simulink model "QuadcopterPID"  (R2024b)
settings: Solver=ode23t  StartTime=0.0  StopTime=path.end_time  FixedStep=0.01  MaxStep=1e-2  RelTol=1e-3  AbsTol=1e-3
undefined symbols (not defined in the file): air_rho, battery_capacity, drone_leg, filtD_motor, filtSpd_motor, kd_motor, ki_motor, kp_motor, limit_motor, max_wind_speed, MPC_config, path, pkgSize, planedepth, qc_motor, qd_area, qd_drag, random_wind, Ts, wind_angle, wind_speed, X, Y, Z
libraries: sm_lib x78, nesl_utility x34, fl_lib x13, slpidlib x9, quadcopter_library x6, ee_lib x4, simulink x4, eeGeneralControl x1, batteryecm_lib x1
(part 1 of 4)
CloseFcn:
  | try,close(h1_quadcopter_package_delivery),end
  | clear h1_quadcopter_package_delivery
  | try,close(h2_quadcopter_package_delivery),end
  | clear h2_quadcopter_package_delivery
  | try,close(h3_quadcopter_package_delivery),end
  | clear h3_quadcopter_package_delivery
  | try,close(h4_quadcopter_package_delivery),end
  | clear h4_quadcopter_package_delivery
Description:
  | Quadcopter Package Delivery
  | Copyright 2021-2024 The MathWorks, Inc.
settings Model: VariantFading=off  Creator=tianwang  LastModifiedBy=danil
settings SolverCC: AutoScaleAbsTol=off  AlgebraicLoopSolver=TrustRegion  SolverResetMethod=Robust
settings DataIOCC: MaxDataPoints=10000  SaveOutput=off  DSMLogging=off  SaveTime=off  ReturnWorkspaceOutputs=off  TimeSaveName=timePID  SignalLoggingName=simPID
settings OptimizationCC: ReuseModelBlockBuffer=off
settings DebuggingCC: ParameterPrecisionLossMsg=none  UnconnectedInputMsg=warning  UnconnectedOutputMsg=warning  UnconnectedLineMsg=warning
settings ModelReferenceCC: EnableRefExpFcnMdlSchedulingChecks=on
settings SFSimCC: CustomCodeUndefinedFunction=UseInterfaceOnly
settings RTWCC: GPUComputeCapability=3.5  DLArmComputeVersion=19.05
settings SimscapeCC: ExplicitSolverDiagnosticOptions=none  SimscapeLogSimulationStatistics=on  SimscapeLogToSDI=on  SimscapeLogName=simlog_quadcopter_package_delivery  SimscapeLogLimitData=off  SimscapeLogDataHistory=50000
settings DiagnosticsConfigSet: SimMechanicsConflictingReferenceFrames=none  SimMechanicsRigidlyBoundBlock=none
settings ExplorerConfigSet: InternalSimMechanicsExplorerSettings="<ExplorerConfiguration><canonicalview>default</canonicalview><AnimationSetting><BasePlaybackSpeed>1.0</BasePlaybackSpeed><PlaybackSpeedFactor>1.0</PlaybackSpeedFactor></AnimationSetting><TilePanel><TileInfo><Tiles Columns=\"2\" Count=\"4\" Rows=\"2\"><Column Weight=\"0.5108\"/><Column Weight=\"0.4892\"/><Row Weight=\"0.4948\"/><Row Weight=\"0.5052\"/><Tile Height=\"1\" Width=\"1\" X=\"0\" Y=\"0\"/><Tile Height=\"1\" Width=\"1\" X=\"0\" Y=\"1\"/><Tile Height=\"1\" Width=\"1\" X=\"1\" Y=\"0\"/><Tile Height=\"1\" Width=\"1\" X=\"1\" Y=\"1\"/></Tiles></TileInfo><SceneInfo><SceneViewer><BGColor><R>1</R><G>1</G><B>1</B></BGColor><Camera><DoPerspective>off</DoPerspective><Position><X>-3.99027915045383441</X><Y>0.687031223743990171</Y><Z>68.9498413117964901</Z></Position><Center><X>-3.99027915045383441</X><Y>0.687031223743990171</Y><Z>3.00000062058594352</Z></Center><Up><X>0</X><Y>1</Y><Z>-0</Z></Up><ViewLimDist>1</ViewLimDist><YLim>5.31135561676258483</YLim><XLim>8.87109395565665793</XLim></Camera></SceneViewer><SceneViewer><BGColor><R>1</R><G>1</G><B>1</B></BGColor><Camera><DoPerspective>on</DoPerspective><Position><X>9.88101233232043086</X><Y>10.0748186090521319</Y><Z>2.02141500533963869</Z></Position><Center><X>9.88101233232043086</X><Y>10.0748186090521319</Y><Z>1.02141500533963869</Z></Center><Up><X>0</X><Y>1</Y><Z>0</Z></Up><ViewLimDist>1</ViewLimDist><YLim>0.466307658154998583</YLim><XLim>0.762607315940987296</XLim></Camera></SceneViewer><SceneViewer><BGColor><R>0.200000002980232239</R><G>0.60000002384185791</G><B>1</B></BGColor><Camera><DoPerspective>on</DoPerspective><Position><X>11.5</X><Y>8.5</Y><Z>1.14000000000000012</Z></Position><Center><X>10</X><Y>10</Y><Z>0.140000000000000013</Z></Center><Up><X>0</X><Y>0</Y><Z>1</Z></Up><ViewLimDist>1</ViewLimDist><YLim>0.466307658154998583</YLim><XLim>0.745761538396823909</XLim></Camera></SceneViewer><SceneViewer><BGColor><R>1</R><G>1</G><B>1</B></BGColor><Camera><DoPerspective>on</DoPerspective><Position><X>10.3810123323204309</X><Y>9.07481860905213189</Y><Z>2.02141500533963869</Z></Position><Center><X>10.0476789989870969</X><Y>9.74148527571879796</Y><Z>1.35474833867297195</Z></Center><Up><X>-0.298142396999971915</X><Y>0.596284793999944052</Y><Z>0.745355992499929787</Z></Up><ViewLimDist>1</ViewLimDist><YLim>0.466307658154998583</YLim><XLim>0.730224839680223559</XLim></Camera></SceneViewer></SceneInfo></TilePanel><MechEditorPanel><Cameras><Camera><Id>Camera1</Id><Value><Name>FixO Top</Name><NativeCamera><PositionTrackingFeature>Quadcopter.Camera.Cam_FixO_Top.R</PositionTrackingFeature><CenterTrackingFeature>Quadcopter.Camera.Cam_FixO_Top.R</CenterTrackingFeature><UpVectorTrackingFeature>Quadcopter.Camera.Cam_FixO_Top.R</UpVectorTrackingFeature><CenterTrackingOrigin>off</CenterTrackingOrigin><CenterTrackingDirection>+X</CenterTrackingDirection><UpVectorTrackingDirection>+Y</UpVectorTrackingDirection></NativeCamera></Value></Camera><Camera><Id>Camera2</Id><Value><Name>FixO L</Name><NativeCamera><PositionTrackingFeature>Quadcopter.Camera.Cam_FixO_L.R</PositionTrackingFeature><CenterTrackingFeature>Quadcopter.Camera.Cam_FixO_L.R</CenterTrackingFeature><UpVectorTrackingFeature>Quadcopter.Camera.Cam_FixO_L.R</UpVectorTrackingFeature><CenterTrackingOrigin>off</CenterTrackingOrigin><CenterTrackingDirection>+X</CenterTrackingDirection><UpVectorTrackingDirection>+Z</UpVectorTrackingDirection></NativeCamera></Value></Camera><Camera><Id>Camera3</Id><Value><Name>FixO F</Name><NativeCamera><PositionTrackingFeature>Quadcopter.Camera.Cam_FixO_F.R</PositionTrackingFeature><CenterTrackingFeature>Quadcopter.Camera.Cam_FixO_F.R</CenterTrackingFeature><UpVectorTrackingFeature>Quadcopter.Camera.Cam_FixO_F.R</UpVectorTrackingFeature><CenterTrackingOrigin>off</CenterTrackingOrigin><CenterTrackingDirection>+X</CenterTrackingDirection><UpVectorTrackingDirection>+Z</UpVectorTrackingDirection></NativeCamera></Value></Camera><Camera><Id>Camera4</Id><Value><Name>FixO UFL</Name><NativeCamera><PositionTrackingFeature>Quadcopter.Camera.Cam_FixO_UFL.R</PositionTrackingFeature><CenterTrackingFeature>Quadcopter.Camera.Cam_FixO_UFL.R</CenterTrackingFeature><UpVectorTrackingFeature>Quadcopter.Camera.Cam_FixO_UFL.R</UpVectorTrackingFeature><CenterTrackingOrigin>off</CenterTrackingOrigin><CenterTrackingDirection>+X</CenterTrackingDirection><UpVectorTrackingDirection>+Z</UpVectorTrackingDirection></NativeCamera></Value></Camera><Camera><Id>Camera5</Id><Value><Name>Track_Target</Name><NativeCamera><PositionTrackingFeature>Quadcopter.Camera.Cam_Target.R</PositionTrackingFeature><CenterTrackingFeature>Quadcopter.Camera.Transform_Target.F</CenterTrackingFeature><UpVectorTrackingFeature>Quadcopter.Camera.Transform_Target.F</UpVectorTrackingFeature><CenterTrackingOrigin>on</CenterTrackingOrigin><UpVectorTrackingDirection>+Z</UpVectorTrackingDirection></NativeCamera></Value></Camera><Camera><Id>Camera6</Id><Value><Name>Track Body Forward</Name><NativeCamera><PositionTrackingFeature>Quadcopter.Body.Body.Cam_Body_Front.R</PositionTrackingFeature><CenterTrackingFeature>Quadcopter.Body.Body.Cam_Body_Front.R</CenterTrackingFeature><UpVectorTrackingFeature>Quadcopter.Body.Body.Cam_Body_Front.R</UpVectorTrackingFeature><CenterTrackingOrigin>off</CenterTrackingOrigin><CenterTrackingDirection>+X</CenterTrackingDirection><UpVectorTrackingDirection>+Z</UpVectorTrackingDirection></NativeCamera></Value></Camera></Cameras><GfxPanelCameraMap><MapElement CameraMLId=\"Camera1\" GfxPanelIndex=\"1\"/><MapElement CameraMLId=\"Camera5\" GfxPanelIndex=\"2\"/><MapElement CameraMLId=\"Camera4\" GfxPanelIndex=\"3\"/></GfxPanelCameraMap><VideoCreator><PlaybackSpeedRatio>1.0</PlaybackSpeedRatio><FrameRate>60</FrameRate><VideoFormat>MPEG-4</VideoFormat><FrameSize>[1920 1080]</FrameSize></VideoCreator></MechEditorPanel></ExplorerConfiguration>"

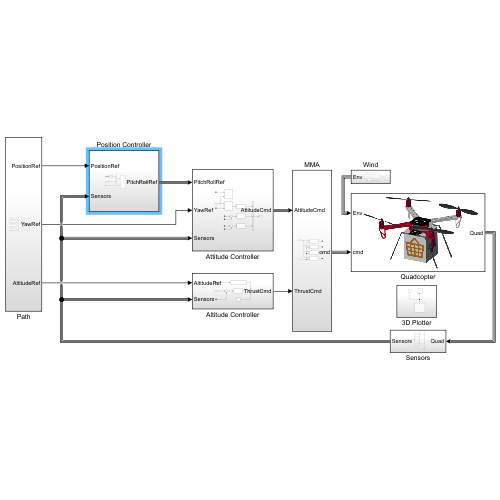
[thumbnail: Simulink's stored preview of the top-level diagram]
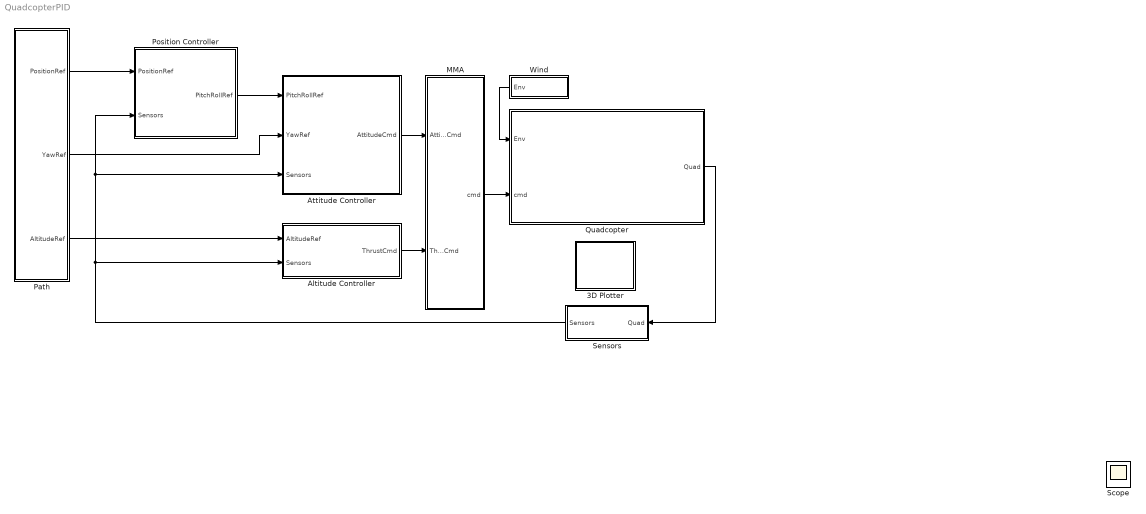
== system QuadcopterPID ==
  3D Plotter : Subsystem
  Altitude Controller : Subsystem
  Attitude Controller : Subsystem
  MMA : Subsystem
  Path : Subsystem
  Position Controller : Subsystem
  Quadcopter : Subsystem
      mask Display:
      | % image('quadcopter_body_arms_load.png');
      | image('quadcopter_body_arms_load_basket.png');
  Sensors : Subsystem
  Wind : Subsystem
  Scope : Scope
  wires:
  Wind/1(Env) -> Quadcopter/1(Env)
  Path/1(PositionRef) -> Position Controller/1(PositionRef)
  Altitude Controller/1(ThrustCmd) -> MMA/2(ThrustCmd)
  MMA/1(cmd) -> Quadcopter/2(cmd)
  Sensors/1(Sensors) -> Position Controller/2(Sensors), Attitude Controller/3(Sensors), Altitude Controller/2(Sensors)
  Path/2(YawRef) -> Attitude Controller/2(YawRef)
  Attitude Controller/1(AttitudeCmd) -> MMA/1(AttitudeCmd)
  Position Controller/1(PitchRollRef) -> Attitude Controller/1(PitchRollRef)
  Path/3(AltitudeRef) -> Altitude Controller/1(AltitudeRef)
  Quadcopter/1(Quad) -> Sensors/1(Quad)

== system QuadcopterPID/3D Plotter ==
  Path : Subsystem
      settings: PortSchema="{\"entries\":[{\"content\":{\"sides\":[{\"content\":{},\"type\":\"ConnectorPlacement.EquallySpacedRectSide\",\"uuid\":\"a37decf6-7c95-4e74-978f-accab4815bca\"},{\"content\":{\"side\":\"RIGHT\"},\"type\":\"ConnectorPlacement.EquallySpacedRectSide\",\"uuid\":\"1290ed2a-5cda-4ac5-b3d1-08d972a37bb4\"},{\"content\":{\"side\":\"TOP\"},\"type\":\"ConnectorPlacement.EquallySpacedRectSide\",\"uuid\":\"57cc8f3c-04dd-443b-a82e-0db9ef1adeeb\"},{\"content\":{\"connectorIds\":[\"RConn1\"],\"side\":\"BOTTOM\"},\"type\":\"ConnectorPlacement.EquallySpacedRectSide\",\"uuid\":\"a98ac24c-8795-4aa4-8cf5-242b040624e5\"}]},\"type\":\"ConnectorPlacement.EquallySpacedConnector\",\"uuid\":\"16016d0d-0355-4838-b6b7-987ac63207fe\"}],\"packageUris\":[\"http://schema.mathworks.com/mf0/Connector/R2020b\"],\"version\":\"1.0\"}"
  Solver Configuration : nesl_utility/Solver Configuration  PhysicalDomain=network_engine_domain  SubClassName=solver  LeftPortType=input  RightPortType=generic  Tones=[]  Harmonics=[]  SimulateNoise=off  Profile=off  UseLocalSampling=off  EnableSwitchedLinearOptims=on  FrequencyDomain=off  UseCCode=off  RelTol=0.001  AbsTol=0.001  MinStep=1e-09  ToWorkspace=off  RevertToSquareIcSolve=off  NumHomotopyIterations=100  PhasorMode=off  PhasorModeNumHarmonics=1  ConsistencySolver=NEWTON_XTOL_AFTER_FTOL  IndexReductionMethod=DerivativeReplacement  DoDC=off  ResidualTolerance=1e-09  ConsistencyTolSource=GLOBAL  ConsistencyAbsTol=0.001  ConsistencyRelTol=0.001  ConsistencyTolFactor=0.001  UseLocalSolver=off  LocalSolverChoice=NE_BACKWARD_EULER_ADVANCER  ResolveIndetEquations=on  FunctionEvalNumThread=1  LocalSolverSampleTime=0.001  DoFixedCost=off  MaxNonlinIter=3  MaxModeIter=2  ComputeImpulses=off  ImpulseIterations=2  LinearAlgebra=auto  LinearAlgebraNumThread=0  EquationFormulation=NE_TIME_EF  DelaysMemoryBudget=1024  AutomaticFiltering=on  FilteringTimeConstant=0.001  PartitionStorageMethod=AS_NEEDED  PartitionMemoryBudget=1024  PartitionMethod=ROBUST  MultibodyUseLocalSolver=off  MultibodyLocalSolverChoice=ODE1  MultibodyLocalSolverSampleTime=0.001
  World Frame : sm_lib/Frames and Transforms/World Frame
  connections:
  World Frame/RConn1 -- Solver Configuration/RConn1 -- Path/RConn1

== system QuadcopterPID/Altitude Controller ==
  AltitudeRef : Inport
  BusElementIn : Inport  Port=2  PortName=Sensors  Element=Position.pz
  BusElementIn1 : Inport  Port=2  PortName=Sensors  Element=LoadStatus
  Constant : Constant  Value=4500
  Control Thrust : slpidlib/PID Controller  Controller=PID  Form=Parallel  TimeDomain=Discrete-time  UseExternalTs=off  SampleTime=-1  IntegratorMethod=Forward Euler  FilterMethod=Forward Euler  ControllerParametersSource=internal  P=2500  I=800  UseKiTs=off  D=3200  UseExternalDerivativeSource=off  N=100  UseFilter=on  TunerSelectOption=Transfer Function Based (PID Tuner App)  ZeroCross=off  InitialConditionSource=internal  InitialConditionForIntegrator=0  InitialConditionForFilter=0  DifferentiatorICPrevScaledInput=0  ExternalReset=none  TrackingMode=off  Kt=1  LimitOutput=on  SatLimitsSource=internal  UpperSaturationLimit=85695  LowerSaturationLimit=-85695  LinearizeAsGain=on  AntiWindupMode=none  Kb=1  LimitIntegrator=off  UpperIntegratorSaturationLimit=inf  LowerIntegratorSaturationLimit=-inf  POutMin=[]  POutMax=[]  IOutMin=[]  IOutMax=[]  DOutMin=[]  DOutMax=[]  NOutMin=[]  NOutMax=[]  SumOutMin=[]  SumOutMax=[]  SaturationOutMin=[]  SaturationOutMax=[]  PParamMin=[]  PParamMax=[]  IParamMin=[]  IParamMax=[]  DParamMin=[]  DParamMax=[]  NParamMin=[]  NParamMax=[]  KbParamMin=[]  KbParamMax=[]  KtParamMin=[]  KtParamMax=[]  KbOutMin=[]  KbOutMax=[]  KtOutMin=[]  KtOutMax=[]  IntegratorOutMin=[]  IntegratorOutMax=[]  FilterOutMin=[]  FilterOutMax=[]  SumI1OutMin=[]  SumI1OutMax=[]  SumI2OutMin=[]  SumI2OutMax=[]  SumI3OutMin=[]  SumI3OutMax=[]  SumI4OutMin=[]  SumI4OutMax=[]  SumDOutMin=[]  SumDOutMax=[]  DifferentiatorOutMin=[]  DifferentiatorOutMax=[]  FilterDiffOutCoefMin=[]  FilterDiffOutCoefMax=[]  ReciprocalOutMin=[]  ReciprocalOutMax=[]  SumDenOutMin=[]  SumDenOutMax=[]  SumNumOutMin=[]  SumNumOutMax=[]  DivideOutMin=[]  DivideOutMax=[]  UdiffTsProdOutMin=[]  UdiffTsProdOutMax=[]  NTsProdOutMin=[]  NTsProdOutMax=[]  UintegralTsProdOutMin=[]  UintegralTsProdOutMax=[]  UngainTsProdOutMin=[]  UngainTsProdOutMax=[]  ClampingZeroOutDataTypeStr=Inherit: Inherit via back propagation  ClampingZeroOutMin=[]  ClampingZeroOutMax=[]  FilterDenConstantOutDataTypeStr=Inherit: Inherit via back propagation  FilterDenConstantOutMin=[]  FilterDenConstantOutMax=[]  PCopyOutDataTypeStr=Inherit: Inherit via back propagation  PCopyOutMin=[]  PCopyOutMax=[]  NCopyOutDataTypeStr=Inherit: Inherit via back propagation  NCopyOutMin=[]  NCopyOutMax=[]  IntegratorContinuousStateAttributes=''  IntegratorStateMustResolveToSignalObject=off  IntegratorRTWStateStorageClass=Auto  FilterContinuousStateAttributes=''  FilterStateMustResolveToSignalObject=off  FilterRTWStateStorageClass=Auto  ParallelPVariant=InternalParameters  IdealPVariant=Disabled  IVariant=InternalParameters  DVariant=InternalParameters  IntegratorVariant=Discrete  SatVariant=Enabled  AWVariant=Passthrough  PCopyVariant=Disabled  TRVariant=Disabled  FdbkBlocksVariant=Forward  IdealPFdbkVariant=Disabled  SatFdbkVariant=Disabled  DerivativeFilterVariant=ForwardEulerFilter  NVariant=InternalParameters  NCopyVariant=Disabled  FilterICVariant=InternalICsFilter  IntegratorICVariant=InternalICs  ExternalResetVariant=Disabled  TRSumVariant=Passthrough  SumFdbkVariant=Disabled  SumVariant=Sum_PID  TsampFilterVariant=InternalTs  TsampNgainVariant=Passthrough  TsampIntegralVariant=Disabled_SignalSpec  ExternalSaturationOutDataTypeStr=Inherit: Same as second input  DerivativeSourceVariant=ErrorSignal  PreIntVariant=InternalPreInt
  Subsystem : Subsystem
  Sum : Sum  Inputs=+++
  Sum1 : Sum  Inputs=|+-
  ThrustCmd : Outport
  wires:
  Sum1/1 -> Control Thrust/1
  BusElementIn/1 -> Sum1/2
  AltitudeRef/1 -> Sum1/1
  Sum/1 -> ThrustCmd/1
  Constant/1 -> Sum/3  "Drone Bias"
  Control Thrust/1 -> Sum/2
  Subsystem/1(Load Bias) -> Sum/1
  BusElementIn1/1 -> Subsystem/1(Load Status)

== system QuadcopterPID/Attitude Controller ==
  Bus Element In1 : Inport  PortName=PitchRollRef
  Bus Element In4 : Inport  PortName=PitchRollRef  Element=pitch
  Bus Element In5 : Inport  PortName=PitchRollRef  Element=roll
  YawRef : Inport  Port=2
  BusElementIn2 : Inport  Port=3  PortName=Sensors  Element=Attitude.roll
  BusElementIn : Inport  Port=3  PortName=Sensors  Element=Attitude.yaw
  BusElementIn1 : Inport  Port=3  PortName=Sensors  Element=Attitude.pitch
  Angle Difference : Subsystem
  Bus Creator : BusCreator  Inputs=3
  Control Pitch : slpidlib/PID Controller  Controller=PID  Form=Parallel  TimeDomain=Discrete-time  UseExternalTs=off  SampleTime=-1  IntegratorMethod=Forward Euler  FilterMethod=Forward Euler  ControllerParametersSource=internal  P=2200  I=3500  UseKiTs=off  D=500  UseExternalDerivativeSource=off  N=100  UseFilter=on  TunerSelectOption=Transfer Function Based (PID Tuner App)  InitialConditionSource=internal  InitialConditionForIntegrator=0  InitialConditionForFilter=0  DifferentiatorICPrevScaledInput=0  ExternalReset=none  TrackingMode=off  Kt=1  LimitOutput=on  SatLimitsSource=internal  UpperSaturationLimit=800  LowerSaturationLimit=-800  LinearizeAsGain=on  AntiWindupMode=clamping  Kb=1  LimitIntegrator=off  UpperIntegratorSaturationLimit=inf  LowerIntegratorSaturationLimit=-inf  POutMin=[]  POutMax=[]  IOutMin=[]  IOutMax=[]  DOutMin=[]  DOutMax=[]  NOutMin=[]  NOutMax=[]  SumOutMin=[]  SumOutMax=[]  SaturationOutMin=[]  SaturationOutMax=[]  PParamMin=[]  PParamMax=[]  IParamMin=[]  IParamMax=[]  DParamMin=[]  DParamMax=[]  NParamMin=[]  NParamMax=[]  KbParamMin=[]  KbParamMax=[]  KtParamMin=[]  KtParamMax=[]  KbOutMin=[]  KbOutMax=[]  KtOutMin=[]  KtOutMax=[]  IntegratorOutMin=[]  IntegratorOutMax=[]  FilterOutMin=[]  FilterOutMax=[]  SumI1OutMin=[]  SumI1OutMax=[]  SumI2OutMin=[]  SumI2OutMax=[]  SumI3OutMin=[]  SumI3OutMax=[]  SumI4OutMin=[]  SumI4OutMax=[]  SumDOutMin=[]  SumDOutMax=[]  DifferentiatorOutMin=[]  DifferentiatorOutMax=[]  FilterDiffOutCoefMin=[]  FilterDiffOutCoefMax=[]  ReciprocalOutMin=[]  ReciprocalOutMax=[]  SumDenOutMin=[]  SumDenOutMax=[]  SumNumOutMin=[]  SumNumOutMax=[]  DivideOutMin=[]  DivideOutMax=[]  UdiffTsProdOutMin=[]  UdiffTsProdOutMax=[]  NTsProdOutMin=[]  NTsProdOutMax=[]  UintegralTsProdOutMin=[]  UintegralTsProdOutMax=[]  UngainTsProdOutMin=[]  UngainTsProdOutMax=[]  ClampingZeroOutDataTypeStr=Inherit: Inherit via back propagation  ClampingZeroOutMin=[]  ClampingZeroOutMax=[]  FilterDenConstantOutDataTypeStr=Inherit: Inherit via back propagation  FilterDenConstantOutMin=[]  FilterDenConstantOutMax=[]  PCopyOutDataTypeStr=Inherit: Inherit via back propagation  PCopyOutMin=[]  PCopyOutMax=[]  NCopyOutDataTypeStr=Inherit: Inherit via back propagation  NCopyOutMin=[]  NCopyOutMax=[]  IntegratorContinuousStateAttributes=''  IntegratorStateMustResolveToSignalObject=off  IntegratorRTWStateStorageClass=Auto  FilterContinuousStateAttributes=''  FilterStateMustResolveToSignalObject=off  FilterRTWStateStorageClass=Auto  ParallelPVariant=InternalParameters  IdealPVariant=Disabled  IVariant=InternalParameters  DVariant=InternalParameters  IntegratorVariant=Discrete  SatVariant=Enabled  AWVariant=DiscClampingParallel  PCopyVariant=Disabled  TRVariant=Disabled  FdbkBlocksVariant=Forward  IdealPFdbkVariant=Disabled  SatFdbkVariant=Disabled  DerivativeFilterVariant=ForwardEulerFilter  NVariant=InternalParameters  NCopyVariant=Disabled  FilterICVariant=InternalICsFilter  IntegratorICVariant=InternalICs  ExternalResetVariant=Disabled  TRSumVariant=Passthrough  SumFdbkVariant=Disabled  SumVariant=Sum_PID  TsampFilterVariant=InternalTs  TsampNgainVariant=Passthrough  TsampIntegralVariant=Disabled_SignalSpec  ExternalSaturationOutDataTypeStr=Inherit: Same as second input  DerivativeSourceVariant=ErrorSignal  PreIntVariant=InternalPreInt
  Control Roll : slpidlib/PID Controller  Controller=PID  Form=Parallel  TimeDomain=Discrete-time  UseExternalTs=off  SampleTime=-1  IntegratorMethod=Forward Euler  FilterMethod=Forward Euler  ControllerParametersSource=internal  P=2200  I=3500  UseKiTs=off  D=500  UseExternalDerivativeSource=off  N=100  UseFilter=on  TunerSelectOption=Transfer Function Based (PID Tuner App)  InitialConditionSource=internal  InitialConditionForIntegrator=0  InitialConditionForFilter=0  DifferentiatorICPrevScaledInput=0  ExternalReset=none  TrackingMode=off  Kt=1  LimitOutput=on  SatLimitsSource=internal  UpperSaturationLimit=800  LowerSaturationLimit=-800  LinearizeAsGain=on  AntiWindupMode=clamping  Kb=1  LimitIntegrator=off  UpperIntegratorSaturationLimit=inf  LowerIntegratorSaturationLimit=-inf  POutMin=[]  POutMax=[]  IOutMin=[]  IOutMax=[]  DOutMin=[]  DOutMax=[]  NOutMin=[]  NOutMax=[]  SumOutMin=[]  SumOutMax=[]  SaturationOutMin=[]  SaturationOutMax=[]  PParamMin=[]  PParamMax=[]  IParamMin=[]  IParamMax=[]  DParamMin=[]  DParamMax=[]  NParamMin=[]  NParamMax=[]  KbParamMin=[]  KbParamMax=[]  KtParamMin=[]  KtParamMax=[]  KbOutMin=[]  KbOutMax=[]  KtOutMin=[]  KtOutMax=[]  IntegratorOutMin=[]  IntegratorOutMax=[]  FilterOutMin=[]  FilterOutMax=[]  SumI1OutMin=[]  SumI1OutMax=[]  SumI2OutMin=[]  SumI2OutMax=[]  SumI3OutMin=[]  SumI3OutMax=[]  SumI4OutMin=[]  SumI4OutMax=[]  SumDOutMin=[]  SumDOutMax=[]  DifferentiatorOutMin=[]  DifferentiatorOutMax=[]  FilterDiffOutCoefMin=[]  FilterDiffOutCoefMax=[]  ReciprocalOutMin=[]  ReciprocalOutMax=[]  SumDenOutMin=[]  SumDenOutMax=[]  SumNumOutMin=[]  SumNumOutMax=[]  DivideOutMin=[]  DivideOutMax=[]  UdiffTsProdOutMin=[]  UdiffTsProdOutMax=[]  NTsProdOutMin=[]  NTsProdOutMax=[]  UintegralTsProdOutMin=[]  UintegralTsProdOutMax=[]  UngainTsProdOutMin=[]  UngainTsProdOutMax=[]  ClampingZeroOutDataTypeStr=Inherit: Inherit via back propagation  ClampingZeroOutMin=[]  ClampingZeroOutMax=[]  FilterDenConstantOutDataTypeStr=Inherit: Inherit via back propagation  FilterDenConstantOutMin=[]  FilterDenConstantOutMax=[]  PCopyOutDataTypeStr=Inherit: Inherit via back propagation  PCopyOutMin=[]  PCopyOutMax=[]  NCopyOutDataTypeStr=Inherit: Inherit via back propagation  NCopyOutMin=[]  NCopyOutMax=[]  IntegratorContinuousStateAttributes=''  IntegratorStateMustResolveToSignalObject=off  IntegratorRTWStateStorageClass=Auto  FilterContinuousStateAttributes=''  FilterStateMustResolveToSignalObject=off  FilterRTWStateStorageClass=Auto  ParallelPVariant=InternalParameters  IdealPVariant=Disabled  IVariant=InternalParameters  DVariant=InternalParameters  IntegratorVariant=Discrete  SatVariant=Enabled  AWVariant=DiscClampingParallel  PCopyVariant=Disabled  TRVariant=Disabled  FdbkBlocksVariant=Forward  IdealPFdbkVariant=Disabled  SatFdbkVariant=Disabled  DerivativeFilterVariant=ForwardEulerFilter  NVariant=InternalParameters  NCopyVariant=Disabled  FilterICVariant=InternalICsFilter  IntegratorICVariant=InternalICs  ExternalResetVariant=Disabled  TRSumVariant=Passthrough  SumFdbkVariant=Disabled  SumVariant=Sum_PID  TsampFilterVariant=InternalTs  TsampNgainVariant=Passthrough  TsampIntegralVariant=Disabled_SignalSpec  ExternalSaturationOutDataTypeStr=Inherit: Same as second input  DerivativeSourceVariant=ErrorSignal  PreIntVariant=InternalPreInt
  Control Yaw : slpidlib/PID Controller  Controller=PID  Form=Parallel  TimeDomain=Discrete-time  UseExternalTs=off  SampleTime=-1  IntegratorMethod=Forward Euler  FilterMethod=Forward Euler  ControllerParametersSource=internal  P=3000  I=1200  UseKiTs=off  D=0  UseExternalDerivativeSource=off  N=100  UseFilter=on  TunerSelectOption=Transfer Function Based (PID Tuner App)  InitialConditionSource=internal  InitialConditionForIntegrator=0  InitialConditionForFilter=0  DifferentiatorICPrevScaledInput=0  ExternalReset=none  TrackingMode=off  Kt=1  LimitOutput=on  SatLimitsSource=internal  UpperSaturationLimit=400  LowerSaturationLimit=-400  LinearizeAsGain=on  AntiWindupMode=clamping  Kb=1  LimitIntegrator=off  UpperIntegratorSaturationLimit=inf  LowerIntegratorSaturationLimit=-inf  POutMin=[]  POutMax=[]  IOutMin=[]  IOutMax=[]  DOutMin=[]  DOutMax=[]  NOutMin=[]  NOutMax=[]  SumOutMin=[]  SumOutMax=[]  SaturationOutMin=[]  SaturationOutMax=[]  PParamMin=[]  PParamMax=[]  IParamMin=[]  IParamMax=[]  DParamMin=[]  DParamMax=[]  NParamMin=[]  NParamMax=[]  KbParamMin=[]  KbParamMax=[]  KtParamMin=[]  KtParamMax=[]  KbOutMin=[]  KbOutMax=[]  KtOutMin=[]  KtOutMax=[]  IntegratorOutMin=[]  IntegratorOutMax=[]  FilterOutMin=[]  FilterOutMax=[]  SumI1OutMin=[]  SumI1OutMax=[]  SumI2OutMin=[]  SumI2OutMax=[]  SumI3OutMin=[]  SumI3OutMax=[]  SumI4OutMin=[]  SumI4OutMax=[]  SumDOutMin=[]  SumDOutMax=[]  DifferentiatorOutMin=[]  DifferentiatorOutMax=[]  FilterDiffOutCoefMin=[]  FilterDiffOutCoefMax=[]  ReciprocalOutMin=[]  ReciprocalOutMax=[]  SumDenOutMin=[]  SumDenOutMax=[]  SumNumOutMin=[]  SumNumOutMax=[]  DivideOutMin=[]  DivideOutMax=[]  UdiffTsProdOutMin=[]  UdiffTsProdOutMax=[]  NTsProdOutMin=[]  NTsProdOutMax=[]  UintegralTsProdOutMin=[]  UintegralTsProdOutMax=[]  UngainTsProdOutMin=[]  UngainTsProdOutMax=[]  ClampingZeroOutDataTypeStr=Inherit: Inherit via back propagation  ClampingZeroOutMin=[]  ClampingZeroOutMax=[]  FilterDenConstantOutDataTypeStr=Inherit: Inherit via back propagation  FilterDenConstantOutMin=[]  FilterDenConstantOutMax=[]  PCopyOutDataTypeStr=Inherit: Inherit via back propagation  PCopyOutMin=[]  PCopyOutMax=[]  NCopyOutDataTypeStr=Inherit: Inherit via back propagation  NCopyOutMin=[]  NCopyOutMax=[]  IntegratorContinuousStateAttributes=''  IntegratorStateMustResolveToSignalObject=off  IntegratorRTWStateStorageClass=Auto  FilterContinuousStateAttributes=''  FilterStateMustResolveToSignalObject=off  FilterRTWStateStorageClass=Auto  ParallelPVariant=InternalParameters  IdealPVariant=Disabled  IVariant=InternalParameters  DVariant=InternalParameters  IntegratorVariant=Discrete  SatVariant=Enabled  AWVariant=DiscClampingParallel  PCopyVariant=Disabled  TRVariant=Disabled  FdbkBlocksVariant=Forward  IdealPFdbkVariant=Disabled  SatFdbkVariant=Disabled  DerivativeFilterVariant=ForwardEulerFilter  NVariant=InternalParameters  NCopyVariant=Disabled  FilterICVariant=InternalICsFilter  IntegratorICVariant=InternalICs  ExternalResetVariant=Disabled  TRSumVariant=Passthrough  SumFdbkVariant=Disabled  SumVariant=Sum_PID  TsampFilterVariant=InternalTs  TsampNgainVariant=Passthrough  TsampIntegralVariant=Disabled_SignalSpec  ExternalSaturationOutDataTypeStr=Inherit: Same as second input  DerivativeSourceVariant=ErrorSignal  PreIntVariant=InternalPreInt
  Data Inspector Plotter : Subsystem
  Sum1 : Sum  Inputs=|+-
  Sum2 : Sum  Inputs=|+-
  AttitudeCmd : Outport
  wires:
  BusElementIn2/1 -> Sum2/2
  Bus Creator/1 -> AttitudeCmd/1
  Bus Element In4/1 -> Sum1/1
  Bus Element In5/1 -> Sum2/1
  YawRef/1 -> Data Inspector Plotter/2(YawRef), Angle Difference/1(YawRef)
  BusElementIn/1 -> Angle Difference/2(Yaw)
  BusElementIn1/1 -> Sum1/2
  Angle Difference/1(Diff) -> Control Yaw/1
  Control Yaw/1 -> Bus Creator/1  "yawCmd"
  Sum1/1 -> Control Pitch/1
  Control Pitch/1 -> Bus Creator/2  "pitchCmd"
  Sum2/1 -> Control Roll/1
  Control Roll/1 -> Bus Creator/3  "rollCmd"
  Bus Element In1/1 -> Data Inspector Plotter/1(PitchRollRef)

== system QuadcopterPID/MMA ==
  AttitudeCmd : Inport
  ThrustCmd : Inport  Port=2
  Calculate w1 : Subsystem
  Calculate w2 : Subsystem
  Calculate w3 : Subsystem
  Calculate w4 : Subsystem
  Bus Element Out : Outport  PortName=cmd  Element=w1
  Bus Element Out1 : Outport  PortName=cmd  Element=w2
  Bus Element Out2 : Outport  PortName=cmd  Element=w3
  Bus Element Out3 : Outport  PortName=cmd  Element=w4
  wires:
  Calculate w1/1(w1) -> Bus Element Out/1
  Calculate w4/1(w4) -> Bus Element Out3/1
  Calculate w3/1(w3) -> Bus Element Out2/1
  Calculate w2/1(w2) -> Bus Element Out1/1
  AttitudeCmd/1 -> Calculate w4/1(AttitudeCmd), Calculate w3/1(AttitudeCmd), Calculate w2/1(AttitudeCmd), Calculate w1/1(AttitudeCmd)
  ThrustCmd/1 -> Calculate w4/2(ThrustCmd), Calculate w3/2(ThrustCmd), Calculate w2/2(ThrustCmd), Calculate w1/2(ThrustCmd)

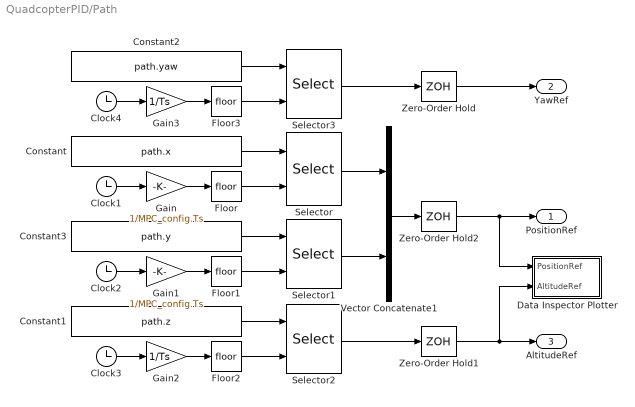
== system QuadcopterPID/Path ==
  Clock{1..4} (4 alike) : Clock
  Constant : Constant  Value=path.x
  Constant1 : Constant  Value=path.z
  Constant2 : Constant  Value=path.yaw
  Constant3 : Constant  Value=path.y
  Data Inspector Plotter : Subsystem
      settings: PortSchema="{\"entries\":[{\"content\":{\"sides\":[{\"content\":{},\"type\":\"ConnectorPlacement.EquallySpacedRectSide\",\"uuid\":\"0f496bf2-b2b6-4bd2-9425-cb84c143776b\"},{\"content\":{\"side\":\"RIGHT\"},\"type\":\"ConnectorPlacement.EquallySpacedRectSide\",\"uuid\":\"68946bc1-57df-4a88-8dd1-ab10ea4e76e5\"},{\"content\":{\"side\":\"TOP\"},\"type\":\"ConnectorPlacement.EquallySpacedRectSide\",\"uuid\":\"57e381a0-7f21-49e7-882a-f855c26e7315\"},{\"content\":{\"connectorIds\":[\"In1\",\"In2\"],\"side\":\"BOTTOM\"},\"type\":\"ConnectorPlacement.EquallySpacedRectSide\",\"uuid\":\"a1114455-6af3-4814-9eeb-f18f60502d18\"}]},\"type\":\"ConnectorPlacement.EquallySpacedConnector\",\"uuid\":\"8716bf71-a1b6-4b1a-bd8c-297568339aba\"}],\"packageUris\":[\"http://schema.mathworks.com/mf0/Connector/R2020b\"],\"version\":\"1.0\"}"
  Floor{,1..3} (4 alike) : Rounding
  Gain : Gain  Gain=1/MPC_config.Ts
  Gain1 : Gain  Gain=1/MPC_config.Ts
  Gain2 : Gain  Gain=1/Ts
  Gain3 : Gain  Gain=1/Ts
  Selector : Selector  IndexMode=Zero-based  InputPortWidth=size(path.x,2)  IndexOptions=Index vector (port)  Indices=[1 3]  OutputSizes=MPC_config.N
  Selector1 : Selector  IndexMode=Zero-based  InputPortWidth=size(path.y,2)  IndexOptions=Index vector (port)  Indices=[1 3]  OutputSizes=MPC_config.N
  Selector2 : Selector  IndexMode=Zero-based  InputPortWidth=size(path.z,2)  IndexOptions=Index vector (port)  Indices=[1 3]  OutputSizes=MPC_config.N
  Selector3 : Selector  IndexMode=Zero-based  InputPortWidth=size(path.yaw,2)  IndexOptions=Index vector (port)  Indices=[1 3]  OutputSizes=MPC_config.N
  Vector Concatenate1 : Concatenate  Mode=Multidimensional array
  Zero-Order Hold : ZeroOrderHold  SampleTime=Ts
  Zero-Order Hold1 : ZeroOrderHold  SampleTime=Ts
  Zero-Order Hold2 : ZeroOrderHold  SampleTime=MPC_config.Ts
  PositionRef : Outport
  YawRef : Outport  Port=2
  AltitudeRef : Outport  Port=3
  wires:
  Clock1/1 -> Gain/1
  Constant/1 -> Selector/1
  Constant3/1 -> Selector1/1
  Gain1/1 -> Floor1/1
  Floor/1 -> Selector/2
  Floor1/1 -> Selector1/2
  Gain/1 -> Floor/1
  Clock2/1 -> Gain1/1
  Clock3/1 -> Gain2/1
  Floor2/1 -> Selector2/2
  Gain2/1 -> Floor2/1
  Constant1/1 -> Selector2/1
  Selector1/1 -> Vector Concatenate1/2
  Selector/1 -> Vector Concatenate1/1
  Constant2/1 -> Selector3/1
  Gain3/1 -> Floor3/1
  Floor3/1 -> Selector3/2
  Clock4/1 -> Gain3/1
  Selector3/1 -> Zero-Order Hold/1
  Vector Concatenate1/1 -> Zero-Order Hold2/1
  Selector2/1 -> Zero-Order Hold1/1
  Zero-Order Hold1/1 -> AltitudeRef/1, Data Inspector Plotter/2(AltitudeRef)
  Zero-Order Hold2/1 -> PositionRef/1, Data Inspector Plotter/1(PositionRef)
  Zero-Order Hold/1 -> YawRef/1

== system QuadcopterPID/Position Controller ==
  PositionRef : Inport
  BusElementIn : Inport  Port=2  PortName=Sensors  Element=Position
  BusElementIn1 : Inport  Port=2  PortName=Sensors  Element=Attitude.yaw
  Bus Creator : BusCreator  Inputs=2
  Bus Selector : BusSelector  OutputSignals=px,py
  Demux : Demux  Outputs=2
  Error : Subsystem
  Low-Pass Filter : eeGeneralControl/Low-Pass Filter (Discrete or Continuous)  K=1  T=0.5  B=inf  A=-inf  init_option=Inherited from block input  x0=0  Ts=Ts
  Mux : Mux  Inputs=2
  PID Controller1 : slpidlib/PID Controller  Controller=PID  Form=Parallel  TimeDomain=Discrete-time  UseExternalTs=off  SampleTime=-1  IntegratorMethod=Forward Euler  FilterMethod=Forward Euler  ControllerParametersSource=internal  P=0.6  I=2  UseKiTs=off  D=1  UseExternalDerivativeSource=off  N=100  UseFilter=on  TunerSelectOption=Transfer Function Based (PID Tuner App)  InitialConditionSource=internal  InitialConditionForIntegrator=0  InitialConditionForFilter=0  DifferentiatorICPrevScaledInput=0  ExternalReset=none  TrackingMode=off  Kt=1  LimitOutput=on  SatLimitsSource=internal  UpperSaturationLimit=MPC_config.limits.pitch  LowerSaturationLimit=-MPC_config.limits.pitch  LinearizeAsGain=on  AntiWindupMode=clamping  Kb=1  LimitIntegrator=off  UpperIntegratorSaturationLimit=inf  LowerIntegratorSaturationLimit=-inf  POutMin=[]  POutMax=[]  IOutMin=[]  IOutMax=[]  DOutMin=[]  DOutMax=[]  NOutMin=[]  NOutMax=[]  SumOutMin=[]  SumOutMax=[]  SaturationOutMin=[]  SaturationOutMax=[]  PParamMin=[]  PParamMax=[]  IParamMin=[]  IParamMax=[]  DParamMin=[]  DParamMax=[]  NParamMin=[]  NParamMax=[]  KbParamMin=[]  KbParamMax=[]  KtParamMin=[]  KtParamMax=[]  KbOutMin=[]  KbOutMax=[]  KtOutMin=[]  KtOutMax=[]  IntegratorOutMin=[]  IntegratorOutMax=[]  FilterOutMin=[]  FilterOutMax=[]  SumI1OutMin=[]  SumI1OutMax=[]  SumI2OutMin=[]  SumI2OutMax=[]  SumI3OutMin=[]  SumI3OutMax=[]  SumI4OutMin=[]  SumI4OutMax=[]  SumDOutMin=[]  SumDOutMax=[]  DifferentiatorOutMin=[]  DifferentiatorOutMax=[]  FilterDiffOutCoefMin=[]  FilterDiffOutCoefMax=[]  ReciprocalOutMin=[]  ReciprocalOutMax=[]  SumDenOutMin=[]  SumDenOutMax=[]  SumNumOutMin=[]  SumNumOutMax=[]  DivideOutMin=[]  DivideOutMax=[]  UdiffTsProdOutMin=[]  UdiffTsProdOutMax=[]  NTsProdOutMin=[]  NTsProdOutMax=[]  UintegralTsProdOutMin=[]  UintegralTsProdOutMax=[]  UngainTsProdOutMin=[]  UngainTsProdOutMax=[]  ClampingZeroOutDataTypeStr=Inherit: Inherit via back propagation  ClampingZeroOutMin=[]  ClampingZeroOutMax=[]  FilterDenConstantOutDataTypeStr=Inherit: Inherit via back propagation  FilterDenConstantOutMin=[]  FilterDenConstantOutMax=[]  PCopyOutDataTypeStr=Inherit: Inherit via back propagation  PCopyOutMin=[]  PCopyOutMax=[]  NCopyOutDataTypeStr=Inherit: Inherit via back propagation  NCopyOutMin=[]  NCopyOutMax=[]  IntegratorContinuousStateAttributes=''  IntegratorStateMustResolveToSignalObject=off  IntegratorRTWStateStorageClass=Auto  FilterContinuousStateAttributes=''  FilterStateMustResolveToSignalObject=off  FilterRTWStateStorageClass=Auto  ParallelPVariant=InternalParameters  IdealPVariant=Disabled  IVariant=InternalParameters  DVariant=InternalParameters  IntegratorVariant=Discrete  SatVariant=Enabled  AWVariant=DiscClampingParallel  PCopyVariant=Disabled  TRVariant=Disabled  FdbkBlocksVariant=Forward  IdealPFdbkVariant=Disabled  SatFdbkVariant=Disabled  DerivativeFilterVariant=ForwardEulerFilter  NVariant=InternalParameters  NCopyVariant=Disabled  FilterICVariant=InternalICsFilter  IntegratorICVariant=InternalICs  ExternalResetVariant=Disabled  TRSumVariant=Passthrough  SumFdbkVariant=Disabled  SumVariant=Sum_PID  TsampFilterVariant=InternalTs  TsampNgainVariant=Passthrough  TsampIntegralVariant=Disabled_SignalSpec  ExternalSaturationOutDataTypeStr=Inherit: Same as second input  DerivativeSourceVariant=ErrorSignal  PreIntVariant=InternalPreInt
  Rate Transition1 : RateTransition  OutPortSampleTime=Ts
  Subtract : Sum  Inputs=-+
  PitchRollRef : Outport
  wires:
  Bus Creator/1 -> PitchRollRef/1
  Bus Selector/1 -> Mux/1  "<px>"
  Bus Selector/2 -> Mux/2  "<py>"
  Mux/1 -> Subtract/1
  Subtract/1 -> Error/1(error_x_y)
  Error/1(error_pitch_roll) -> PID Controller1/1
  Demux/2 -> Bus Creator/2  "roll"
  PID Controller1/1 -> Low-Pass Filter/1
  PositionRef/1 -> Rate Transition1/1
  BusElementIn/1 -> Bus Selector/1
  BusElementIn1/1 -> Error/2(Yaw)
  Rate Transition1/1 -> Subtract/2
  Low-Pass Filter/1 -> Demux/1
  Demux/1 -> Bus Creator/1  "pitch"

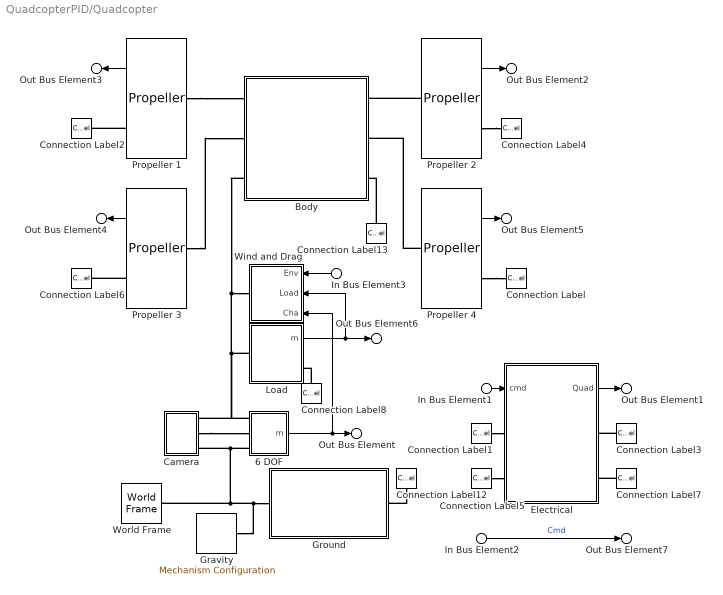
== system QuadcopterPID/Quadcopter ==
  In Bus Element3 : Inport  PortName=Env  Element=wind
  In Bus Element1 : Inport  Port=2  PortName=cmd
  In Bus Element2 : Inport  Port=2  PortName=cmd
  6 DOF : Subsystem
  Body : Subsystem
      mask Display: image('quadcopter_body_arms.png');
  Camera : Subsystem
  Connection Label : ConnectionLabel  Label=P4
  Connection Label1 : ConnectionLabel  Label=P4
  Connection Label12 : ConnectionLabel  Label=G
  Connection Label13 : ConnectionLabel  Label=G
  Connection Label2 : ConnectionLabel  Label=P1
  Connection Label3 : ConnectionLabel  Label=P1
  Connection Label4 : ConnectionLabel  Label=P2
  Connection Label5 : ConnectionLabel  Label=P2
  Connection Label6 : ConnectionLabel  Label=P3
  Connection Label7 : ConnectionLabel  Label=P3
  Connection Label8 : ConnectionLabel  Label=G
  Electrical : Subsystem  mask{trq_max=qc_motor.max_torque, power_max=qc_motor.max_power, trq_tc=qc_motor.time_const, eff_overall=qc_motor.efficiency, eff_spd=qc_motor.efficiency_spd, eff_trq=qc_motor.efficiency_trq, rotor_d=qc_motor.rotor_damping, kp=kp_motor, ki=ki_motor, kd=kd_motor, f_deriv=filtD_motor, f_spd=filtSpd_motor, max_trq_cmd=limit_motor}
      mask prompts: trq_max "Max Torque (N*m)"; power_max "Max Power (W)"; trq_tc "Time Constant, Torque (s)"; eff_overall "Efficiency (%)"; eff_spd "Speed for Efficiency (rpm)"; eff_trq "Torque for Efficiency (N*m)"; rotor_d "Rotor Damping (N*m/(rad/s))"; kp "Proportional"; ki "Integral"; kd "Derivative"; f_deriv "Filter on Error Derivative (N)"; f_spd "Filter on Speed Measurement (sec)"; max_trq_cmd "Saturation (N*m)"
      mask DialogControl Container4 Prompt: Motor
      mask DialogControl Container9 Prompt: Control
      mask Display: image('quadcopter_electric.png');
  Gravity : sm_lib/Utilities/Mechanism Configuration  UniformGravity=Constant  GravityVector=[0 0 -9.80665]  GravityVectorUnits=m/s^2  LinearizationDelta=0.001  JointModeTransitionNonlinearIterations=2
  Ground : Subsystem
      mask Display: image('ground_launch_target.PNG');
  Load : Subsystem
      mask Display:
      | %image('medical_kit.png');
      | image('load_package_basket.png');
  Propeller 1 : quadcopter_library/Propeller  popup_prop_pos=1 or 4
  Propeller 2 : quadcopter_library/Propeller  popup_prop_pos=2 or 3
  Propeller 3 : quadcopter_library/Propeller  popup_prop_pos=2 or 3
  Propeller 4 : quadcopter_library/Propeller  popup_prop_pos=1 or 4
  Wind and Drag : Subsystem
  World Frame : sm_lib/Frames and Transforms/World Frame
  Out Bus Element : Outport  PortName=Quad  Element=Chassis
  Out Bus Element1 : Outport  PortName=Quad  Element=Motor
  Out Bus Element2 : Outport  PortName=Quad  Element=Prop2
  Out Bus Element3 : Outport  PortName=Quad  Element=Prop1
  Out Bus Element4 : Outport  PortName=Quad  Element=Prop3
  Out Bus Element5 : Outport  PortName=Quad  Element=Prop4
  Out Bus Element6 : Outport  PortName=Quad  Element=Load
  Out Bus Element7 : Outport  PortName=Quad  Element=cmd
  wires:
  Propeller 4/1 -> Out Bus Element5/1
  Propeller 1/1 -> Out Bus Element3/1
  Propeller 3/1 -> Out Bus Element4/1
  Electrical/1(Quad) -> Out Bus Element1/1
  Propeller 2/1 -> Out Bus Element2/1
  In Bus Element1/1 -> Electrical/1(cmd)
  6 DOF/1(m) -> Out Bus Element/1, Wind and Drag/3(Cha)
  Load/1(m) -> Out Bus Element6/1, Wind and Drag/2(Load)
  In Bus Element3/1 -> Wind and Drag/1(Env)
  In Bus Element2/1 -> Out Bus Element7/1  "Cmd"
  connections:
  Body/LConn3 -- 6 DOF/LConn1 -- Camera/RConn1 -- Load/LConn1 -- Wind and Drag/RConn1
  Propeller 2/LConn1 -- Body/RConn1
  Propeller 1/LConn1 -- Body/LConn1
  Propeller 4/LConn1 -- Body/RConn2
  Propeller 3/LConn1 -- Body/LConn2
  Connection Label13/LConn1 -- Body/RConn3
  Propeller 4/RConn1 -- Connection Label/LConn1
  Connection Label1/LConn1 -- Electrical/LConn1
  Propeller 1/RConn1 -- Connection Label2/LConn1
  Connection Label3/LConn1 -- Electrical/RConn1
  Propeller 2/RConn1 -- Connection Label4/LConn1
  Connection Label5/LConn1 -- Electrical/LConn2
  Propeller 3/RConn1 -- Connection Label6/LConn1
  Connection Label7/LConn1 -- Electrical/RConn2
  Gravity/RConn1 -- 6 DOF/LConn3 -- Camera/RConn3 -- World Frame/RConn1 -- Ground/RConn1
  Connection Label12/LConn1 -- Ground/LConn1
  Connection Label8/LConn1 -- Load/RConn1
  Camera/RConn2 -- 6 DOF/LConn2

== system QuadcopterPID/Sensors ==
  Quad : Inport
  Bias : Bias  Bias=1  SaturateOnIntegerOverflow=off
  Bus Creator : BusCreator  Inputs=3
  Bus Creator1 : BusCreator  Inputs=3
  Bus Creator2 : BusCreator  Inputs=4
  Bus Creator3 : BusCreator  Inputs=3
  Bus Selector : BusSelector  OutputSignals=Chassis.px,Chassis.py,Chassis.pz,Chassis.yaw,Chassis.pitch,Chassis.roll,Chassis.ax,Chassis.ay,Chassis.az,Load.status
  Zero-Order Hold : ZeroOrderHold  SampleTime=Ts
  Sensors : Outport
  wires:
  Quad/1 -> Zero-Order Hold/1  "Quadcopter"
  Bus Selector/2 -> Bus Creator/2  "<py>"
  Bus Selector/3 -> Bus Creator/3  "<pz>"
  Bus Selector/1 -> Bus Creator/1  "<px>"
  Bus Selector/4 -> Bus Creator1/1  "<yaw>"
  Bus Selector/5 -> Bus Creator1/2  "<pitch>"
  Bus Selector/6 -> Bus Creator1/3  "<roll>"
  Bus Creator1/1 -> Bus Creator2/2  "Attitude"
  Bus Creator/1 -> Bus Creator2/1  "Position"
  Bus Creator2/1 -> Sensors/1  "Sensors"
  Zero-Order Hold/1 -> Bus Selector/1
  Bus Selector/7 -> Bus Creator3/1  "<ax>"
  Bus Selector/8 -> Bus Creator3/2  "<ay>"
  Bus Selector/9 -> Bus Creator3/3  "<az>"
  Bus Creator3/1 -> Bus Creator2/3  "Acceleration"
  Bias/1 -> Bus Creator2/4  "LoadStatus"
  Bus Selector/10 -> Bias/1  "<status>"

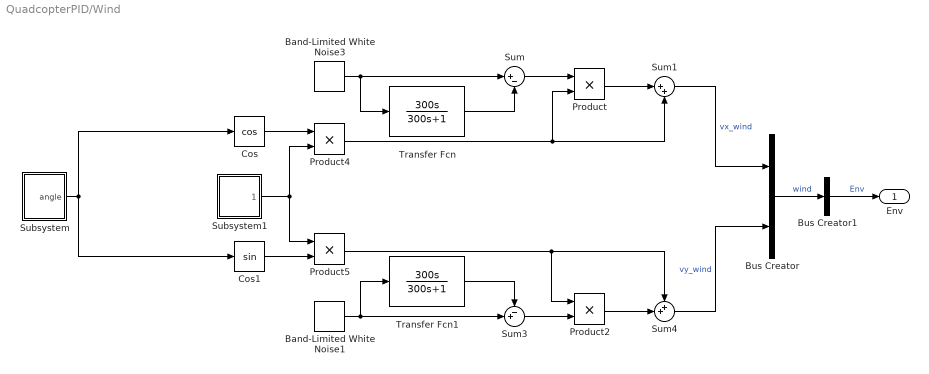
== system QuadcopterPID/Wind ==
  Band-Limited White Noise1 : simulink/Sources/Band-Limited White Noise  Cov=[0.1]  Ts=0.1  seed=[23341]
  Band-Limited White Noise3 : simulink/Sources/Band-Limited White Noise  Cov=[0.1]  Ts=0.1  seed=[23341]
  Bus Creator : BusCreator  Inputs=2
  Bus Creator1 : BusCreator  Inputs=1
  Cos : Trigonometry  Operator=cos
  Cos1 : Trigonometry
  Product{,2,4..5} (4 alike) : Product
  Subsystem : Subsystem
  Subsystem1 : Subsystem
  Sum : Sum  Inputs=|+-
  Sum1 : Sum  Inputs=|++
  Sum3 : Sum  Inputs=-+|
  Sum4 : Sum  Inputs=++|
  Transfer Fcn : TransferFcn  Numerator=[300 0]  Denominator=[300 1]
  Transfer Fcn1 : TransferFcn  Numerator=[300 0]  Denominator=[300 1]
  Env : Outport
  wires:
  Product4/1 -> Sum1/2, Product/2
  Transfer Fcn/1 -> Sum/2
  Sum/1 -> Product/1
  Band-Limited White Noise3/1 -> Sum/1, Transfer Fcn/1
  Product/1 -> Sum1/1
  Bus Creator/1 -> Bus Creator1/1  "wind"
  Bus Creator1/1 -> Env/1  "Env"
  Cos/1 -> Product4/1
  Subsystem1/1(speed) -> Product5/1, Product4/2
  Cos1/1 -> Product5/2
  Product2/1 -> Sum4/2
  Product5/1 -> Product2/1, Sum4/1
  Transfer Fcn1/1 -> Sum3/1
  Band-Limited White Noise1/1 -> Sum3/2, Transfer Fcn1/1
  Sum3/1 -> Product2/2
  Sum1/1 -> Bus Creator/1  "vx_wind"
  Sum4/1 -> Bus Creator/2  "vy_wind"
  Subsystem/1(angle) -> Cos1/1, Cos/1

== system QuadcopterPID/3D Plotter/Path ==
  Spline1 : sm_lib/Curves and Surfaces/Spline  DataPoints=unique([path.x' path.y' path.z(round(linspace(1,size(path.z,2),size(path.x,2))))'],'rows','stable')  DataPointsUnits=m  EndConditionType=Natural  GraphicType=FromGeometry  MarkerShape=Frame  MarkerSize=10  GraphicVisPropType=SimpleVisualProperties  GraphicDiffuseColor=[1 1 0]  GraphicOpacity=0.2  GraphicSpecularColor=[0.5 0.5 0.5 1.0]  GraphicAmbientColor=[0.15 0.15 0.15 1.0]  GraphicEmissiveColor=[0.0 0.0 0.0 1.0]  GraphicShininess=75
  W : PMIOPort  Side=Right
  connections:
  Spline1/LConn1 -- W/RConn1

== system QuadcopterPID/Altitude Controller/Subsystem ==
  Bus Element In1 : Inport  PortName=Load Status
  Constant1 : Constant  Value=1500
  Constant2 : Constant  Value=0
  Switch : Switch  Criteria=u2 > Threshold  SaturateOnIntegerOverflow=off  InputSameDT=off
  Load Bias : Outport
  wires:
  Switch/1 -> Load Bias/1
  Bus Element In1/1 -> Switch/2
  Constant1/1 -> Switch/1
  Constant2/1 -> Switch/3

== system QuadcopterPID/Attitude Controller/Angle Difference ==
  YawRef : Inport
  Yaw : Inport  Port=2
  Bias : Bias  Bias=pi  SaturateOnIntegerOverflow=off
  Bias1 : Bias  Bias=-pi  SaturateOnIntegerOverflow=off
  Bias2 : Bias  Bias=2*pi  SaturateOnIntegerOverflow=off
  Constant : Constant  Value=2*pi
  Mod : Math  Operator=mod
  Sum : Sum  Inputs=|+-
  Switch : Switch  Criteria=u2 > Threshold  Threshold=-pi  SaturateOnIntegerOverflow=off  InputSameDT=off
  Diff : Outport
  wires:
  YawRef/1 -> Sum/1
  Yaw/1 -> Sum/2
  Sum/1 -> Bias/1
  Bias/1 -> Mod/1
  Constant/1 -> Mod/2
  Mod/1 -> Bias1/1
  Bias1/1 -> Bias2/1, Switch/1, Switch/2
  Bias2/1 -> Switch/3
  Switch/1 -> Diff/1

== system QuadcopterPID/Attitude Controller/Data Inspector Plotter ==
  Bus Element In1 : Inport  PortName=PitchRollRef
  YawRef : Inport  Port=2
  Bus Creator : BusCreator  Inputs=3
  Bus Selector : BusSelector  OutputSignals=pitch,roll
  Terminator : Terminator
  wires:
  Bus Element In1/1 -> Bus Selector/1
  Bus Selector/1 -> Bus Creator/2  "<pitch>"
  Bus Selector/2 -> Bus Creator/3  "<roll>"
  YawRef/1 -> Bus Creator/1  "yaw"
  Bus Creator/1 -> Terminator/1  "AttitudeRef"

== system QuadcopterPID/MMA/Calculate w1 ==
  AttitudeCmd : Inport
  ThrustCmd : Inport  Port=2
  Bus Selector : BusSelector  OutputSignals=yawCmd,pitchCmd,rollCmd
  Subtract : Sum  Inputs=--++
  w1 : Outport
  wires:
  AttitudeCmd/1 -> Bus Selector/1
  Bus Selector/2 -> Subtract/2  "<pitchCmd>"
  Bus Selector/3 -> Subtract/3  "<rollCmd>"
  Bus Selector/1 -> Subtract/1  "<yawCmd>"
  ThrustCmd/1 -> Subtract/4
  Subtract/1 -> w1/1

== system QuadcopterPID/MMA/Calculate w2 ==
  AttitudeCmd : Inport
  ThrustCmd : Inport  Port=2
  Bus Selector : BusSelector  OutputSignals=yawCmd,pitchCmd,rollCmd
  Subtract : Sum  Inputs=+--+
  w2 : Outport
  wires:
  Subtract/1 -> w2/1
  ThrustCmd/1 -> Subtract/4
  AttitudeCmd/1 -> Bus Selector/1
  Bus Selector/3 -> Subtract/3  "<rollCmd>"
  Bus Selector/2 -> Subtract/2  "<pitchCmd>"
  Bus Selector/1 -> Subtract/1  "<yawCmd>"

== system QuadcopterPID/MMA/Calculate w3 ==
  AttitudeCmd : Inport
  ThrustCmd : Inport  Port=2
  Bus Selector : BusSelector  OutputSignals=yawCmd,pitchCmd,rollCmd
  Subtract : Sum  Inputs=++++
  w3 : Outport
  wires:
  Subtract/1 -> w3/1
  ThrustCmd/1 -> Subtract/4
  AttitudeCmd/1 -> Bus Selector/1
  Bus Selector/3 -> Subtract/3  "<rollCmd>"
  Bus Selector/2 -> Subtract/2  "<pitchCmd>"
  Bus Selector/1 -> Subtract/1  "<yawCmd>"

== system QuadcopterPID/MMA/Calculate w4 ==
  AttitudeCmd : Inport
  ThrustCmd : Inport  Port=2
  Bus Selector : BusSelector  OutputSignals=yawCmd,pitchCmd,rollCmd
  Subtract : Sum  Inputs=-+-+
  w4 : Outport
  wires:
  Subtract/1 -> w4/1
  ThrustCmd/1 -> Subtract/4
  AttitudeCmd/1 -> Bus Selector/1
  Bus Selector/3 -> Subtract/3  "<rollCmd>"
  Bus Selector/2 -> Subtract/2  "<pitchCmd>"
  Bus Selector/1 -> Subtract/1  "<yawCmd>"

== system QuadcopterPID/Path/Data Inspector Plotter ==
  PositionRef : Inport
  AltitudeRef : Inport  Port=2
  Bus Creator : BusCreator  Inputs=3
  Demux : Demux  Outputs=2
  Terminator1 : Terminator
  wires:
  PositionRef/1 -> Demux/1
  Demux/1 -> Bus Creator/1  "x"
  Demux/2 -> Bus Creator/2  "y"
  AltitudeRef/1 -> Bus Creator/3  "z"
  Bus Creator/1 -> Terminator1/1  "Path"

== system QuadcopterPID/Position Controller/Error ==
  error_x_y : Inport
  Yaw : Inport  Port=2
  Atan2 : Trigonometry  Operator=atan2
  Cos : Trigonometry  Operator=cos
  Demux : Demux  Outputs=2
  Gain : Gain  Gain=-1
  Mux : Mux  Inputs=2
  Norm : Subsystem
  Product : Product
  Product1 : Product
  Sin : Trigonometry
  Sum : Sum  Inputs=|+-
  error_pitch_roll : Outport
  wires:
  Atan2/1 -> Sum/1
  Yaw/1 -> Sum/2
  Sum/1 -> Sin/1, Cos/1
  Cos/1 -> Product/2
  Norm/1(norm) -> Product1/2, Product/1
  Sin/1 -> Product1/1
  Product1/1 -> Gain/1
  error_x_y/1 -> Norm/1(error), Demux/1
  Demux/2 -> Atan2/1
  Demux/1 -> Atan2/2
  Mux/1 -> error_pitch_roll/1
  Product/1 -> Mux/1
  Gain/1 -> Mux/2
